simulink model "gm_MyRegModel_Simulink"  (R2023b)
settings: Solver=FixedStepDiscrete  StartTime=0.0  StopTime=50  RelTol=1e-3
undefined symbols (not defined in the file or in its folder): t0, t1, t2, t3, t4, t5
libraries: dspsrcs4 x6
settings Model: Creator=ravir  LastModifiedBy=ravir
settings OptimizationCC: BlockReduction=off  ConditionallyExecuteInputs=off  DefaultParameterBehavior=Inlined  InheritOutputTypeSmallerThanSingle=on
settings DebuggingCC: AlgebraicLoopMsg=error  InheritedTsInSrcMsg=none  SingleTaskRateTransMsg=error  ParameterOverflowMsg=none  ParameterPrecisionLossMsg=none
settings HardwareCC: ProdBitPerPointer=32  ProdBitPerSizeT=32  ProdBitPerPtrDiffT=32  ProdLargestAtomicFloat=None  ProdIntDivRoundTo=Undefined  ProdEndianess=Unspecified  ProdWordSize=32  ProdHWDeviceType=ASIC/FPGA->ASIC/FPGA  TargetBitPerPointer=64  TargetBitPerSizeT=64  TargetBitPerPtrDiffT=64  TargetLongLongMode=on  TargetIntDivRoundTo=Zero  TargetEndianess=LittleEndian  TargetWordSize=64  TargetHWDeviceType=Custom Processor->MATLAB Host Computer  ProdEqTarget=off

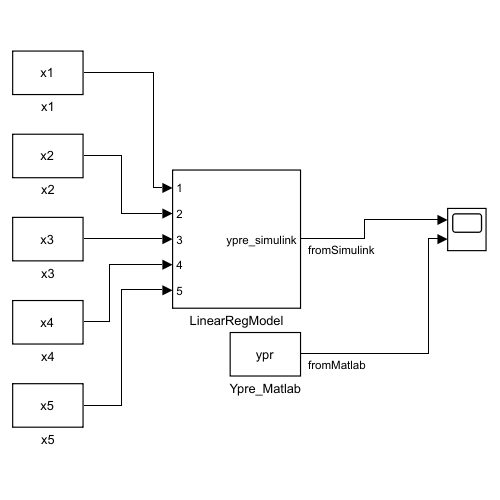
[thumbnail: Simulink's stored preview of the top-level diagram]
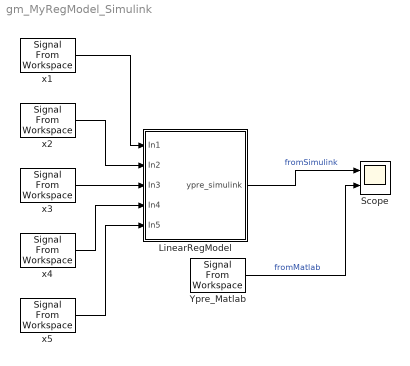
== system gm_MyRegModel_Simulink ==
  LinearRegModel : Subsystem
  Scope : Scope  NumInputPorts=2
  Ypre_Matlab : dspsrcs4/Signal From Workspace  X=ypr  Ts=1  nsamps=1  OutputAfterFinalValue=Setting to zero  ignoreOrWarnInputAndFrameLengths=off  OutputFrames=off
  x1 : dspsrcs4/Signal From Workspace  X=x1  Ts=1  nsamps=1  OutputAfterFinalValue=Setting to zero  ignoreOrWarnInputAndFrameLengths=off  OutputFrames=off
  x2 : dspsrcs4/Signal From Workspace  X=x2  Ts=1  nsamps=1  OutputAfterFinalValue=Setting to zero  ignoreOrWarnInputAndFrameLengths=off  OutputFrames=off
  x3 : dspsrcs4/Signal From Workspace  X=x3  Ts=1  nsamps=1  OutputAfterFinalValue=Setting to zero  ignoreOrWarnInputAndFrameLengths=off  OutputFrames=off
  x4 : dspsrcs4/Signal From Workspace  X=x4  Ts=1  nsamps=1  OutputAfterFinalValue=Setting to zero  ignoreOrWarnInputAndFrameLengths=off  OutputFrames=off
  x5 : dspsrcs4/Signal From Workspace  X=x5  Ts=1  nsamps=1  OutputAfterFinalValue=Setting to zero  ignoreOrWarnInputAndFrameLengths=off  OutputFrames=off
  wires:
  LinearRegModel/1(ypre_simulink) -> Scope/1  "fromSimulink"
  x5/1 -> LinearRegModel/5(In5)
  Ypre_Matlab/1 -> Scope/2  "fromMatlab"
  x4/1 -> LinearRegModel/4(In4)
  x2/1 -> LinearRegModel/2(In2)
  x3/1 -> LinearRegModel/3(In3)
  x1/1 -> LinearRegModel/1(In1)

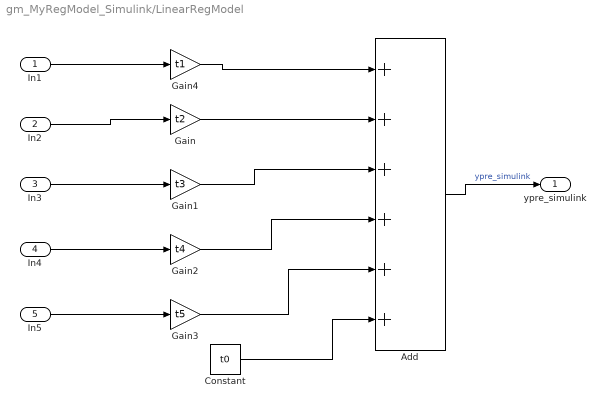
== system gm_MyRegModel_Simulink/LinearRegModel ==
  In1 : Inport
  In2 : Inport  Port=2
  In3 : Inport  Port=3
  In4 : Inport  Port=4
  In5 : Inport  Port=5
  Add : Sum  Inputs=++++++  OutDataTypeStr=fixdt(0,24,3)
  Constant : Constant  Value=t0  VectorParams1D=off  OutDataTypeStr=fixdt(1,32,9)  SampleTime=-1
  Gain : Gain  Gain=t2
  Gain1 : Gain  Gain=t3
  Gain2 : Gain  Gain=t4
  Gain3 : Gain  Gain=t5
  Gain4 : Gain  Gain=t1
  ypre_simulink : Outport
  wires:
  Constant/1 -> Add/6
  In3/1 -> Gain1/1
  In4/1 -> Gain2/1
  In1/1 -> Gain4/1
  In5/1 -> Gain3/1
  Add/1 -> ypre_simulink/1  "ypre_simulink"
  Gain1/1 -> Add/3
  Gain3/1 -> Add/5
  Gain2/1 -> Add/4
  In2/1 -> Gain/1
  Gain4/1 -> Add/1
  Gain/1 -> Add/2
